simulink model "Constant_TestGen36"  (R2017b)
settings: Solver=FixedStepDiscrete  StartTime=0.0  StopTime=10.0  RelTol=1e-3
undefined symbols (not defined in the file): Block_TestLib, enable_trigger
settings Model: Creator=ktrinh  LastModifiedBy=hbourbou
settings DebuggingCC: ParameterOverflowMsg=none

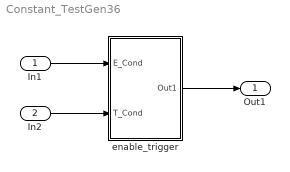
== system Constant_TestGen36 ==
  In1 : Inport
  In2 : Inport  Port=2
  enable_trigger : Subsystem  AncestorBlock=Block_TestLib/enable_trigger
  Out1 : Outport
  wires:
  In1/1 -> enable_trigger/1(E_Cond)
  In2/1 -> enable_trigger/2(T_Cond)
  enable_trigger/1(Out1) -> Out1/1

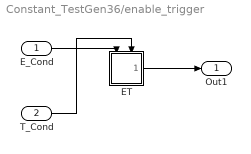
== system Constant_TestGen36/enable_trigger ==
  E_Cond : Inport  OutDataTypeStr=boolean
  T_Cond : Inport  Port=2  OutDataTypeStr=boolean
  ET : Subsystem  TreatAsAtomicUnit=on
  Out1 : Outport
  wires:
  T_Cond/1 -> ET/Trigger
  E_Cond/1 -> ET/Enable
  ET/1(Out1) -> Out1/1

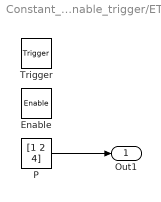
== system Constant_TestGen36/enable_trigger/ET ==
  Enable : EnablePort
  Trigger : TriggerPort  VariantControl=Variant
  P : Constant  Value=[1 2 4]  OutDataTypeStr=uint32
  Out1 : Outport  InitialOutput=3
  wires:
  P/1 -> Out1/1
